simulink library "time"  (R2021b)
settings: Solver=VariableStepAuto  StartTime=0.0  StopTime=10.0  RelTol=1e-3
libraries: simulink x3
settings Model: Creator=Davide  LastModifiedBy=Davide

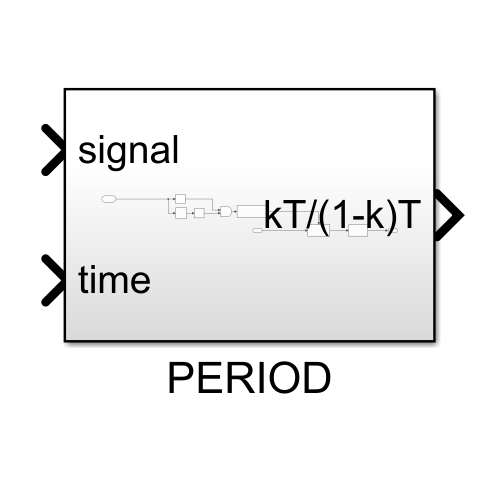
[thumbnail: Simulink's stored preview of the top-level diagram]
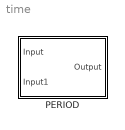
== system time ==
  PERIOD : Subsystem

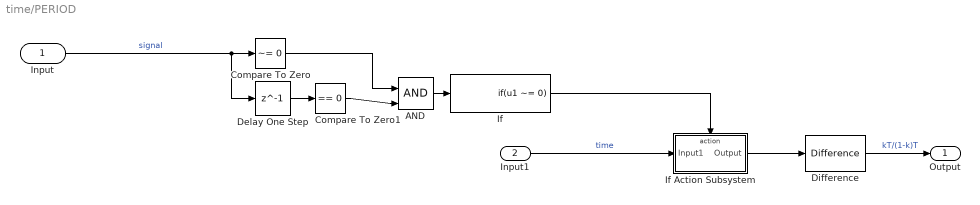
== system time/PERIOD ==
  Input : Inport
  Input1 : Inport  Port=2
  AND : Logic  IconShape=distinctive  AllPortsSameDT=off  OutDataTypeStr=boolean
  Compare To Zero : simulink/Logic and Bit Operations/Compare To Zero  relop=~=  OutDataTypeStr=boolean
  Compare To Zero1 : simulink/Logic and Bit Operations/Compare To Zero  relop===  OutDataTypeStr=boolean
  Delay One Step : Delay  DelayLength=1
  Difference : simulink/Discrete/Difference  ICPrevInput=0.0  OutMin=[]  OutMax=[]  OutDataType=fixdt(1, 16)  OutScaling=2^-10  DoSatur=off
  If : If  IfExpression=u1 ~= 0  ShowElse=off
  If Action Subsystem : Subsystem  TreatAsAtomicUnit=on
  Output : Outport
  wires:
  Input/1 -> Delay One Step/1, Compare To Zero/1  "signal"
  AND/1 -> If/1
  Input1/1 -> If Action Subsystem/1(Input1)  "time"
  Compare To Zero1/1 -> AND/2
  Compare To Zero/1 -> AND/1
  If Action Subsystem/1(Output) -> Difference/1
  If/1 -> If Action Subsystem/Action
  Delay One Step/1 -> Compare To Zero1/1
  Difference/1 -> Output/1  "kT/(1-k)T"

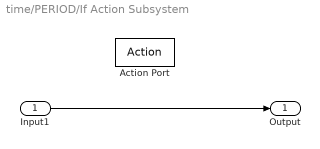
== system time/PERIOD/If Action Subsystem ==
  Input1 : Inport
  Action Port : ActionPort  ActionPortLabel=if(u1 > 0)
  Output : Outport
  wires:
  Input1/1 -> Output/1
